simulink model "bp5_model2"  (R2019b)
settings: Solver=ode45  StartTime=0.0  StopTime=10.0  RelTol=1e-12  AbsTol=1e-12
PreLoadFcn:
  | ww=[1e-9 1e7]; N=59;
undefined symbols (not defined in the file or in its folder): G
libraries: cstblocks x3
settings Model: Creator=Professor Dingyu Xue  LastModifiedBy=xuedi
settings SolverCC: AutoScaleAbsTol=off
settings DataIOCC: SaveFormat=Array  ReturnWorkspaceOutputs=off
settings DebuggingCC: ArithmeticOperatorsInVariantConditions=warning
settings SFSimCC: SimUseLocalCustomCode=off  CustomCodeUndefinedFunction=UseInterfaceOnly
settings RTWCC: RTWUseLocalCustomCode=off
settings CodeAppCC: StateflowObjectComments=on

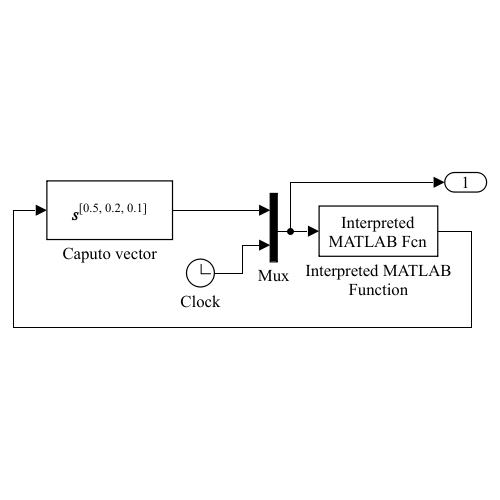
[thumbnail: Simulink's stored preview of the top-level diagram]
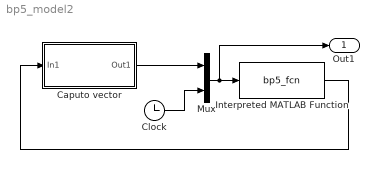
== system bp5_model2 ==
  Caputo vector : Subsystem  mask{gam=[0.5 0.2 0.1], ww=ww, N=N, M=3, x0=[1 0.5 0.3]}
      mask prompts: gam "Derivative order gamma"; ww "Frequency range [wb,wh]"; N "Apprixmation order N"; M "Dimension M"; x0 "Initial condition x0"
      mask init:
      | wb=ww(1); wh=ww(2); stri=[];
      |    if length(gam)==1, gam=gam*ones(M,1); end
      |    for i=1:M
      |       G(i,1)=ousta_fod(1-gam(i),N,wb,wh); stri=[stri,num2str(gam(i)),', '];
      |    end
      |    str=['{\bf{\its}}^{[' stri(1:end-2) ']}'];
      |    svec2sl(gam);
      mask Display: disp(str,'texmode','on')
  Clock : Clock
  Interpreted MATLAB Function : MATLABFcn  MATLABFcn=bp5_fcn  OutputDimensions=3
  Mux : Mux  Inputs=2
  Out1 : Outport
  wires:
  Mux/1 -> Out1/1, Interpreted MATLAB Function/1
  Clock/1 -> Mux/2
  Caputo vector/1(Out1) -> Mux/1
  Interpreted MATLAB Function/1 -> Caputo vector/1(In1)

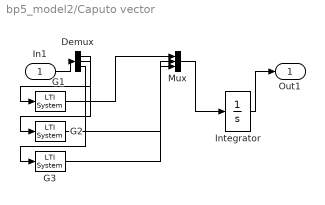
== system bp5_model2/Caputo vector ==
  In1 : Inport
  Demux : Demux  Outputs=3
  G1 : cstblocks/LTI System  sys=G(1)  IC=[]
  G2 : cstblocks/LTI System  sys=G(2)  IC=[]
  G3 : cstblocks/LTI System  sys=G(3)  IC=[]
  Integrator : Integrator  InitialCondition=x0
  Mux : Mux  Inputs=3
  Out1 : Outport
  wires:
  Demux/1 -> G1/1
  G1/1 -> Mux/1
  Demux/2 -> G2/1
  G2/1 -> Mux/2
  Demux/3 -> G3/1
  G3/1 -> Mux/3
  Integrator/1 -> Out1/1
  Mux/1 -> Integrator/1
  In1/1 -> Demux/1
